simulink model "RC_LinearInterpolation"  (R2018a)
settings: Solver=FixedStepAuto  StartTime=0.0  StopTime=0.5  FixedStep=1e-4  RelTol=1e-3
InitFcn:
  | Ts = 1e-4
  | fg = 49.2
libraries: powerlib_meascontrol x1
settings Model: Creator=donghao  LastModifiedBy=donghao
settings CodeAppCC: StateflowObjectComments=on
settings SimscapeCC: SimscapeNormalizeSystem=off

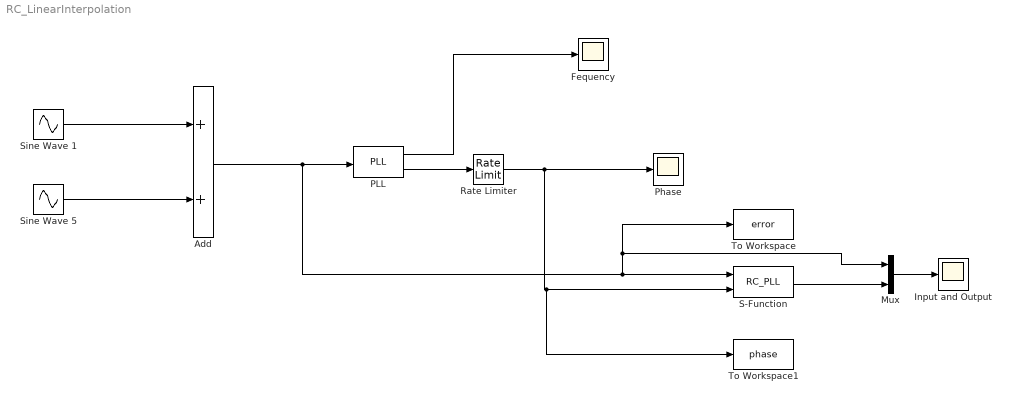
== system RC_LinearInterpolation ==
  Add : Sum
  Fequency : Scope
  Input and Output : Scope
  Mux : Mux  Inputs=2
  PLL : powerlib_meascontrol/PLL/PLL  Fmin=49.5  Par_Init=[0, 50]  ParK=[180, 3200, 1]  TcD=1e-4  MaxRateChangeFreq=12  FilterCutOffFreq=25  Ts=0  AGC=on
      settings: SourceProductName=Simscape Power Systems  SourceProductBaseCode=PS
  Phase : Scope
  Rate Limiter : RateLimiter  RisingSlewLimit=400  FallingSlewLimit=-1e10  SampleTimeMode=inherited
  S-Function : S-Function  FunctionName=RC_PLL  SFunctionDeploymentMode=off  EnableBusSupport=off
  Sine Wave 1 : Sin  Frequency=2 * pi * fg  SampleTime=Ts
  Sine Wave 5 : Sin  Amplitude=0.1  Frequency=2 * pi * fg * 5  SampleTime=Ts
  To Workspace : ToWorkspace  VariableName=error  SampleTime=1e-4
      settings: Save2DSignal=2-D array (concatenate along first dimension)
  To Workspace1 : ToWorkspace  VariableName=phase  SampleTime=1e-4
      settings: Save2DSignal=2-D array (concatenate along first dimension)
  wires:
  PLL/1 -> Fequency/1
  Mux/1 -> Input and Output/1
  Sine Wave 1/1 -> Add/1
  Add/1 -> To Workspace/1, Mux/1, S-Function/1, PLL/1
  Sine Wave 5/1 -> Add/2
  S-Function/1 -> Mux/2
  PLL/2 -> Rate Limiter/1
  Rate Limiter/1 -> To Workspace1/1, S-Function/2, Phase/1
